simulink model "VehV_VD"  (R2016b)
settings: configuration reference "CodeGenConfigSet" (kept outside this file)
values from neighbouring files (symbols this model uses):
  SigTst_nCrdSh_C = Calibration.Parameter    [init_VehV_VD.m]
  SigTst_swtCrDSh = Calibration.Parameter    [init_VehV_VD.m]
  SigTst_swtVehV = Calibration.Parameter    [init_VehV_VD.m]
  SigTst_vVehV_C = Calibration.Parameter    [init_VehV_VD.m]
  VehV_facAPT1_C = Calibration.Parameter    [init_VehV_VD.m]
  VehV_facNCrdShPT1_C = Calibration.Parameter    [init_VehV_VD.m]
  VehV_facVPT1_C = Calibration.Parameter    [init_VehV_VD.m]
  VehV_nCrdShDfl_C = Calibration.Parameter    [init_VehV_VD.m]
  VehV_nMinCrdSh_C = Calibration.Parameter    [init_VehV_VD.m]
  VehV_nThresPla_C = Calibration.Parameter    [init_VehV_VD.m]
  VehV_swtTrqSel_C = Calibration.Parameter    [init_VehV_VD.m]
  VehV_tiDebMonPla_C = Calibration.Parameter    [init_VehV_VD.m]
  VehV_trqThresPla_C = Calibration.Parameter    [init_VehV_VD.m]
  VehV_vDfl_C = Calibration.Parameter    [init_VehV_VD.m]
  VehV_vMax_C = Calibration.Parameter    [init_VehV_VD.m]
  VehV_vMin_C = Calibration.Parameter    [init_VehV_VD.m]
  VehV_vThresPla_C = Calibration.Parameter    [init_VehV_VD.m]
undefined symbols (not defined in the file or in its folder): Switch_conv, VehV_VD_DT
libraries: CXLib x6, simulink x1
settings Model: Creator=胡炎林  LastModifiedBy=lenovo
settings ConfigSetRef: SourceLocation=Base Workspace

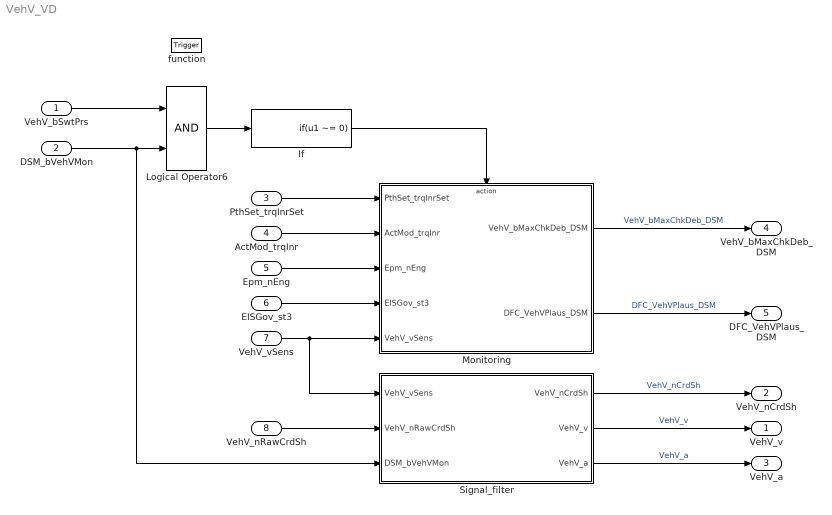
== system VehV_VD ==
  VehV_bSwtPrs : Inport  Description=sensor switch  OutMin=0  OutMax=1  OutDataTypeStr=boolean
  DSM_bVehVMon : Inport  Description=state of FId_VehVMon  Port=2  OutMin=0  OutMax=1  OutDataTypeStr=boolean
  PthSet_trqInrSet : Inport  Tag=Nm  Description=Inner torque set value after monitoring limitation  Port=3  OutMin=-3000  OutMax=3276.7  OutDataTypeStr=Trq_Nm
  ActMod_trqInr : Inport  Tag=Nm  Description=Current, back-calculated inner engine torque  Port=4  OutMin=-3276.8  OutMax=3276.7  OutDataTypeStr=Trq_Nm
  Epm_nEng : Inport  Tag=rpm  Description=Engine speed  Port=5  OutMin=0  OutMax=6000  OutDataTypeStr=EngSpeed_rpm
  EISGov_st3 : Inport  Description=Status information of WESDem client  Port=6  OutMin=0  OutMax=2147483648  OutDataTypeStr=State_uint32
  VehV_vSens : Inport  Tag=km/h  Description=Sensed vehicle speed  Port=7  OutMin=0  OutMax=250  OutDataTypeStr=VehSpeed_km_h
  VehV_nRawCrdSh : Inport  Tag=rpm  Description=Raw Cardan shaft speed  Port=8  OutMin=0  OutMax=6000  OutDataTypeStr=EngSpeed_rpm
  function : TriggerPort  TriggerType=function-call  VariantControl=Variant
  If : If  IfExpression=u1 ~= 0  ShowElse=off
  Logical Operator6 : Logic  OutDataTypeStr=boolean
  Monitoring : Subsystem
  Signal_filter : Subsystem
  VehV_v : Outport  Tag=km/h  Description=Vehicle speed  OutMin=0  OutMax=250  OutDataTypeStr=VehSpeed_km_h
  VehV_nCrdSh : Outport  Tag=rpm  Description=Cardan shaft speed  Port=2  OutMin=0  OutMax=6000  OutDataTypeStr=EngSpeed_rpm
  VehV_a : Outport  Tag=m/s^2  Description=The acceleration of the vehicle  Port=3  OutMin=-32.7  OutMax=32.7  OutDataTypeStr=Acc_m_s2
  VehV_bMaxChkDeb_DSM : Outport  Description=status of VehV_bMaxChkDeb  Port=4  OutMin=0  OutMax=1  OutDataTypeStr=boolean
  DFC_VehVPlaus_DSM : Outport  Description=state of DFC_VehVPlaus  Port=5  OutMin=0  OutMax=1  OutDataTypeStr=boolean
  wires:
  Signal_filter/2(VehV_v) -> VehV_v/1  "VehV_v"
  Signal_filter/1(VehV_nCrdSh) -> VehV_nCrdSh/1  "VehV_nCrdSh"
  Signal_filter/3(VehV_a) -> VehV_a/1  "VehV_a"
  VehV_bSwtPrs/1 -> Logical Operator6/1
  Logical Operator6/1 -> If/1
  VehV_nRawCrdSh/1 -> Signal_filter/2(VehV_nRawCrdSh)
  VehV_vSens/1 -> Monitoring/5(VehV_vSens), Signal_filter/1(VehV_vSens)
  EISGov_st3/1 -> Monitoring/4(EISGov_st3)
  Epm_nEng/1 -> Monitoring/3(Epm_nEng)
  ActMod_trqInr/1 -> Monitoring/2(ActMod_trqInr)
  PthSet_trqInrSet/1 -> Monitoring/1(PthSet_trqInrSet)
  DSM_bVehVMon/1 -> Signal_filter/3(DSM_bVehVMon), Logical Operator6/2
  If/1 -> Monitoring/Action
  Monitoring/1(VehV_bMaxChkDeb_DSM) -> VehV_bMaxChkDeb_DSM/1  "VehV_bMaxChkDeb_DSM"
  Monitoring/2(DFC_VehVPlaus_DSM) -> DFC_VehVPlaus_DSM/1  "DFC_VehVPlaus_DSM"

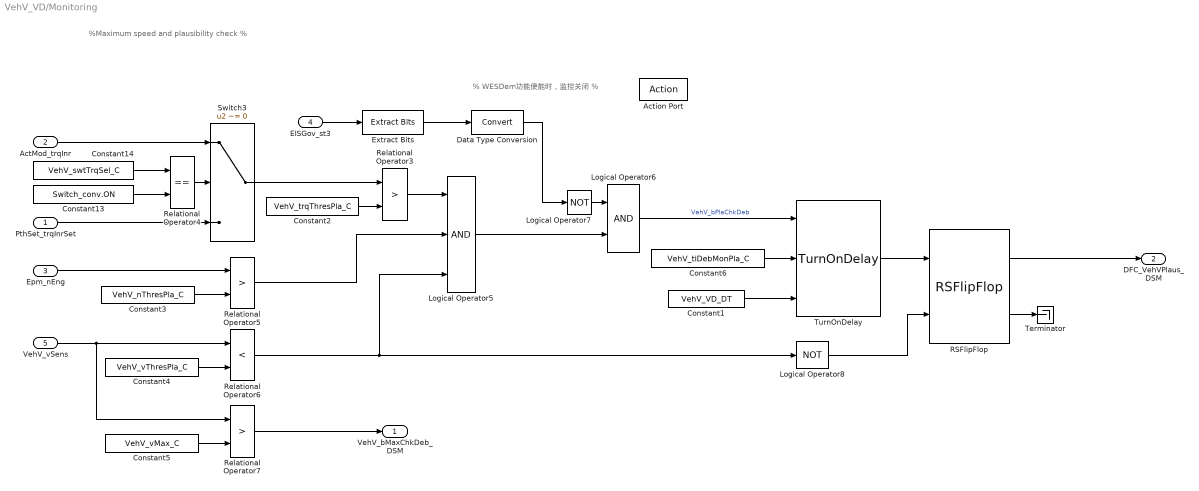
== system VehV_VD/Monitoring ==
  note: %Maximum speed and plausibility check %
  note: % WESDem功能使能时，监控关闭 %
  PthSet_trqInrSet : Inport
  ActMod_trqInr : Inport  Port=2
  Epm_nEng : Inport  Port=3
  EISGov_st3 : Inport  Port=4
  VehV_vSens : Inport  Port=5
  Action Port : ActionPort  ActionType=then
  Constant1 : Constant  Value=VehV_VD_DT
  Constant13 : Constant  Value=Switch_conv.ON  OutDataTypeStr=Inherit: Inherit via back propagation
  Constant14 : Constant  Value=VehV_swtTrqSel_C
  Constant2 : Constant  Value=VehV_trqThresPla_C
  Constant3 : Constant  Value=VehV_nThresPla_C
  Constant4 : Constant  Value=VehV_vThresPla_C
  Constant5 : Constant  Value=VehV_vMax_C
  Constant6 : Constant  Value=VehV_tiDebMonPla_C
  Data Type Conversion : DataTypeConversion
  Extract Bits : simulink/Logic and Bit Operations/Extract Bits  bitsToExtract=Range of bits  numBits=8  bitIdxRange=7  outScalingMode=Preserve fixed-point scaling
  Logical Operator5 : Logic  Inputs=3  OutDataTypeStr=boolean
  Logical Operator6 : Logic  OutDataTypeStr=boolean
  Logical Operator7 : Logic  Operator=NOT  OutDataTypeStr=boolean
  Logical Operator8 : Logic  Operator=NOT  OutDataTypeStr=boolean
  RSFlipFlop : CXLib/RSFlipFlop
  Relational Operator3 : RelationalOperator  Operator=>  OutDataTypeStr=boolean  RndMeth=Nearest  InputSameDT=on
  Relational Operator4 : RelationalOperator  Operator===  OutDataTypeStr=boolean  RndMeth=Nearest  InputSameDT=on
  Relational Operator5 : RelationalOperator  Operator=>  OutDataTypeStr=boolean  RndMeth=Nearest  InputSameDT=on
  Relational Operator6 : RelationalOperator  Operator=<  OutDataTypeStr=boolean  RndMeth=Nearest  InputSameDT=on
  Relational Operator7 : RelationalOperator  Operator=>  OutDataTypeStr=boolean  RndMeth=Nearest  InputSameDT=on
  Switch3 : Switch  Criteria=u2 ~= 0  InputSameDT=on
  Terminator : Terminator
  TurnOnDelay : CXLib/TurnOnDelay
  VehV_bMaxChkDeb_DSM : Outport
  DFC_VehVPlaus_DSM : Outport  Port=2
  wires:
  Constant5/1 -> Relational Operator7/2
  Logical Operator6/1 -> TurnOnDelay/1  "VehV_bPlaChkDeb"
  RSFlipFlop/2 -> Terminator/1
  TurnOnDelay/1 -> RSFlipFlop/1
  Constant6/1 -> TurnOnDelay/2
  Logical Operator8/1 -> RSFlipFlop/2
  RSFlipFlop/1 -> DFC_VehVPlaus_DSM/1
  Relational Operator7/1 -> VehV_bMaxChkDeb_DSM/1
  Logical Operator7/1 -> Logical Operator6/1
  EISGov_st3/1 -> Extract Bits/1
  Logical Operator5/1 -> Logical Operator6/2
  Relational Operator6/1 -> Logical Operator5/3, Logical Operator8/1
  Constant4/1 -> Relational Operator6/2
  VehV_vSens/1 -> Relational Operator6/1, Relational Operator7/1
  Relational Operator5/1 -> Logical Operator5/2
  Epm_nEng/1 -> Relational Operator5/1
  Constant3/1 -> Relational Operator5/2
  Relational Operator3/1 -> Logical Operator5/1
  Constant2/1 -> Relational Operator3/2
  Switch3/1 -> Relational Operator3/1
  PthSet_trqInrSet/1 -> Switch3/3
  ActMod_trqInr/1 -> Switch3/1
  Relational Operator4/1 -> Switch3/2
  Constant13/1 -> Relational Operator4/2
  Constant14/1 -> Relational Operator4/1
  Constant1/1 -> TurnOnDelay/3
  Extract Bits/1 -> Data Type Conversion/1
  Data Type Conversion/1 -> Logical Operator7/1

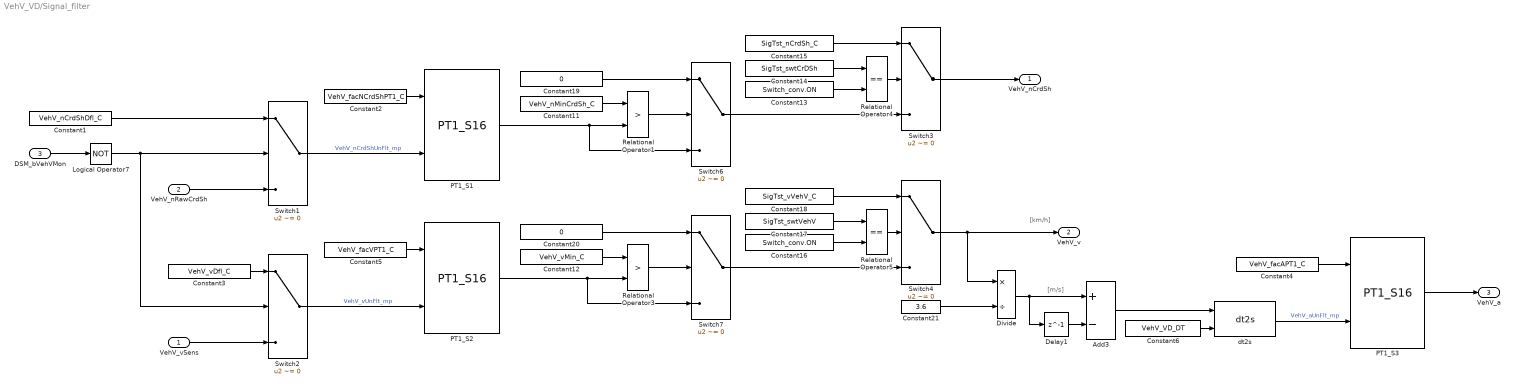
== system VehV_VD/Signal_filter ==
  note: [m/s]
  note: [km/h]
  VehV_vSens : Inport
  VehV_nRawCrdSh : Inport  Port=2
  DSM_bVehVMon : Inport  Description=state of FId_VehVMon  Port=3  OutMin=0  OutMax=1  OutDataTypeStr=boolean
  Add3 : Sum  Inputs=+-  OutDataTypeStr=Inherit: Inherit via back propagation  SaturateOnIntegerOverflow=on  InputSameDT=on
  Constant1 : Constant  Value=VehV_nCrdShDfl_C  SampleTime=-1
  Constant11 : Constant  Value=VehV_nMinCrdSh_C  SampleTime=-1
  Constant12 : Constant  Value=VehV_vMin_C  SampleTime=-1
  Constant13 : Constant  Value=Switch_conv.ON  OutDataTypeStr=Inherit: Inherit via back propagation
  Constant14 : Constant  Value=SigTst_swtCrDSh
  Constant15 : Constant  Value=SigTst_nCrdSh_C
  Constant16 : Constant  Value=Switch_conv.ON  OutDataTypeStr=Inherit: Inherit via back propagation
  Constant17 : Constant  Value=SigTst_swtVehV
  Constant18 : Constant  Value=SigTst_vVehV_C
  Constant19 : Constant  Value=0  OutDataTypeStr=Inherit: Inherit via back propagation  SampleTime=-1
  Constant2 : Constant  Value=VehV_facNCrdShPT1_C  SampleTime=-1
  Constant20 : Constant  Value=0  OutDataTypeStr=Inherit: Inherit via back propagation  SampleTime=-1
  Constant21 : Constant  Value=3.6  OutDataTypeStr=fixdt(1,16,2)
  Constant3 : Constant  Value=VehV_vDfl_C  SampleTime=-1
  Constant4 : Constant  Value=VehV_facAPT1_C  SampleTime=-1
  Constant5 : Constant  Value=VehV_facVPT1_C  SampleTime=-1
  Constant6 : Constant  Value=VehV_VD_DT
  Delay1 : Delay  DelayLength=1  InitialCondition=0
  Divide : Product  Inputs=*/  OutDataTypeStr=Inherit: Inherit via back propagation
  Logical Operator7 : Logic  Operator=NOT  OutDataTypeStr=boolean
  PT1_S1 : CXLib/PT1_S16
  PT1_S2 : CXLib/PT1_S16
  PT1_S3 : CXLib/PT1_S16
  Relational Operator1 : RelationalOperator  Operator=>  OutDataTypeStr=boolean  RndMeth=Nearest  InputSameDT=on
  Relational Operator3 : RelationalOperator  Operator=>  OutDataTypeStr=boolean  RndMeth=Nearest  InputSameDT=on
  Relational Operator4 : RelationalOperator  Operator===  OutDataTypeStr=boolean  RndMeth=Nearest  InputSameDT=on
  Relational Operator5 : RelationalOperator  Operator===  OutDataTypeStr=boolean  RndMeth=Nearest  InputSameDT=on
  Switch{1..4,6..7} (6 alike) : Switch  Criteria=u2 ~= 0  InputSameDT=on
  dt2s : CXLib/dt2s
  VehV_nCrdSh : Outport
  VehV_v : Outport  Port=2
  VehV_a : Outport  Port=3
  wires:
  Add3/1 -> dt2s/1
  Delay1/1 -> Add3/2
  Divide/1 -> Delay1/1, Add3/1
  Constant21/1 -> Divide/2
  dt2s/1 -> PT1_S3/2  "VehV_aUnFlt_mp"
  Constant4/1 -> PT1_S3/1
  VehV_vSens/1 -> Switch2/3
  Constant3/1 -> Switch2/1
  VehV_nRawCrdSh/1 -> Switch1/3
  Constant1/1 -> Switch1/1
  DSM_bVehVMon/1 -> Logical Operator7/1
  Logical Operator7/1 -> Switch1/2, Switch2/2
  PT1_S3/1 -> VehV_a/1
  Switch4/1 -> Divide/1, VehV_v/1
  Switch3/1 -> VehV_nCrdSh/1
  Switch7/1 -> Switch4/3
  Constant20/1 -> Switch7/1
  Switch6/1 -> Switch3/3
  Constant19/1 -> Switch6/1
  Relational Operator3/1 -> Switch7/2
  Constant18/1 -> Switch4/1
  Relational Operator5/1 -> Switch4/2
  Constant16/1 -> Relational Operator5/2
  Constant17/1 -> Relational Operator5/1
  Relational Operator1/1 -> Switch6/2
  Constant15/1 -> Switch3/1
  Relational Operator4/1 -> Switch3/2
  Constant13/1 -> Relational Operator4/2
  Constant14/1 -> Relational Operator4/1
  Constant6/1 -> dt2s/2
  PT1_S2/1 -> Relational Operator3/2, Switch7/3
  Constant12/1 -> Relational Operator3/1
  Constant11/1 -> Relational Operator1/1
  PT1_S1/1 -> Relational Operator1/2, Switch6/3
  Constant5/1 -> PT1_S2/1
  Switch1/1 -> PT1_S1/2  "VehV_nCrdShUnFlt_mp"
  Constant2/1 -> PT1_S1/1
  Switch2/1 -> PT1_S2/2  "VehV_vUnFlt_mp"
